simulink model "reconstruct_albatros_dual_15"  (R2021a)
settings: Solver=VariableStepAuto  StartTime=0.0  StopTime=10.0  RelTol=1e-3
undefined symbols (not defined in the file): pfb_coeff_gen_calc
libraries: xbsIndex_r4 x5175, casper_library_misc x31, casper_library_delays x24, xps_library x4
(part 16 of 71)

== system reconstruct_albatros_dual_15/tvg0/tvg ==
  addr : Inport
  data_in : Inport  Port=2
  we : Inport  Port=3
  Terminator : Terminator
  Terminator1 : Terminator
  Terminator2 : Terminator
  calc_add : Subsystem  mask{data_width=64, addr_width=12, sample_rate=sample_rate}
      mask prompts: data_width "data width"; addr_width "address width"; sample_rate "sample rate"
  convert_addr : xbsIndex_r4/Convert  gui_display_data_type=Fixed-point  arith_type=Unsigned  n_bits=addr_width  bin_pt=0  float_type=Single  exp_bits=8  fraction_bits=24  quantization=Truncate  overflow=Wrap  en=off  latency=0  pipeline=off  dbl_ovrd=off  block_type=convert
      settings: xl_area=[0, 0, 0, 0, 0, 0, 0]
  convert_din1 : xbsIndex_r4/Convert  gui_display_data_type=Fixed-point  arith_type=Unsigned  n_bits=64  bin_pt=0  float_type=Single  exp_bits=8  fraction_bits=24  quantization=Truncate  overflow=Wrap  en=off  latency=0  pipeline=off  dbl_ovrd=off  block_type=convert
      settings: xl_area=[0, 0, 0, 0, 0, 0, 0]
  convert_we : xbsIndex_r4/Convert  gui_display_data_type=Fixed-point  arith_type=Unsigned  n_bits=1  bin_pt=0  float_type=Single  exp_bits=8  fraction_bits=24  quantization=Truncate  overflow=Wrap  en=off  latency=0  pipeline=off  dbl_ovrd=off  block_type=convert
      settings: xl_area=[0, 0, 0, 0, 0, 0, 0]
  munge_in : Subsystem  AncestorBlock=casper_library_flow_control/munge  mask(munge){divisions=2, div_size=[32 32], order=[1  0], arith_type_out=Unsigned, bin_pt_out=0}
      mask prompts: divisions "Number of divisions"; div_size "Division size (bits)"; order "Division packing order"; arith_type_out "Output arithmetic type"; bin_pt_out "Output binary point"
      mask help: Splits an input bus into the specified number of divisions and then recombines them in the order specified (most significant division = 0,least = number divisions-1)
      mask init:
      | munge_init(gcb, ...
      |     'divisions', divisions, ...
      |     'div_size', div_size, ...
      |     'order', order, ...
      |     'arith_type_out', arith_type_out, ...
      |     'bin_pt_out', bin_pt_out);
      settings: AttributesFormatString=|
      | split:[32 32]
      | join:[1 0]
      | Unsigned [64,0]
      mask TypeOptions arith_type_out: Unsigned | Signed  (2's comp) | Floating-point
  munge_out : Subsystem  AncestorBlock=casper_library_flow_control/munge  mask(munge){divisions=2, div_size=[32 32], order=[1  0], arith_type_out=Unsigned, bin_pt_out=0}
      mask prompts: divisions "Number of divisions"; div_size "Division size (bits)"; order "Division packing order"; arith_type_out "Output arithmetic type"; bin_pt_out "Output binary point"
      mask help: Splits an input bus into the specified number of divisions and then recombines them in the order specified (most significant division = 0,least = number divisions-1)
      mask init:
      | munge_init(gcb, ...
      |     'divisions', divisions, ...
      |     'div_size', div_size, ...
      |     'order', order, ...
      |     'arith_type_out', arith_type_out, ...
      |     'bin_pt_out', bin_pt_out);
      settings: AttributesFormatString=|
      | split:[32 32]
      | join:[1 0]
      | Unsigned [64,0]
      mask TypeOptions arith_type_out: Unsigned | Signed  (2's comp) | Floating-point
  reconstruct_albatros_dual_15_tvg0_tvg_addr : xbsIndex_r4/Gateway Out  inherit_from_input=off  hdl_port=on  rows=1  columns=1  UseAsDAC=off  DACChannel='1'  interface=None  automatic_assignment=on  address_offset=hex2dec('00')  intf_name=''  intf_description=''  timing_constraint=None  locs_specified=off  LOCs={'A5','B9','A9','C1','A3','G6','E9','A6','A7','A8','B8','B1','B3','D9','B5','B4','B6','C2'}  io_standard={}  block_type=gatewayout
      settings: infoedit="Gateway out block.  Converts Xilinx fixed point inputs into ouputs of type Simulink integer, double, or fixed point.<P><P>Hardware notes:  In hardware these blocks become top level output ports or are discarded, depending on how they are configured."  sginterface={'Nallatech'=>{'xdspkit'=>{'non_memory_mapped_port'=>'uprev_Shared_BRAM_addr'}},'Xilinx'=>{'jtaghwcosim'=>{'non_memory_mapped_port'=>'uprev_Shared_BRAM_addr'},'xdspkit'=>{'non_memory_mapped_port'=>'uprev_Shared_BRAM_addr'}}}  xl_area=[0, 0, 0, 0, 0, 0, 0]
  reconstruct_albatros_dual_15_tvg0_tvg_data_in : xbsIndex_r4/Gateway Out  inherit_from_input=off  hdl_port=on  rows=1  columns=1  UseAsDAC=off  DACChannel='1'  interface=None  automatic_assignment=on  address_offset=hex2dec('00')  intf_name=''  intf_description=''  timing_constraint=None  locs_specified=off  LOCs={'B21','B22','A22','B23','B19','C19','A20','A21','A23','B24','A24','A25','E18','D18','C18','B18'}  io_standard={}  block_type=gatewayout
      settings: infoedit="Gateway out block.  Converts Xilinx fixed point inputs into ouputs of type Simulink integer, double, or fixed point.<P><P>Hardware notes:  In hardware these blocks become top level output ports or are discarded, depending on how they are configured."  sginterface={'Nallatech'=>{'xdspkit'=>{'non_memory_mapped_port'=>'uprev_Shared_BRAM_data_in'}},'Xilinx'=>{'jtaghwcosim'=>{'non_memory_mapped_port'=>'uprev_Shared_BRAM_data_in'},'xdspkit'=>{'non_memory_mapped_port'=>'uprev_Shared_BRAM_data_in'}}}  xl_area=[0, 0, 0, 0, 0, 0, 0]
  reconstruct_albatros_dual_15_tvg0_tvg_data_out : xbsIndex_r4/Gateway In  gui_display_data_type=Fixed-point  arith_type=Unsigned  n_bits=64  bin_pt=0  preci_type=Single  exp_width=8  frac_width=24  rows=1  columns=1  quantization=Truncate  overflow=Wrap  period=sample_rate  UseAsADC=off  ADCChannel='1'  interface=None  automatic_assignment=on  address_offset=hex2dec('00')  intf_name=''  intf_description=''  default_value=0  timing_constraint=None  locs_specified=off  LOCs={}  io_standard={}  inherit_from_input=off  hdl_port=on  dbl_ovrd=off  block_type=gatewayin
      settings: xl_area=[0, 0, 0, 0, 0, 0, 0]
  reconstruct_albatros_dual_15_tvg0_tvg_we : xbsIndex_r4/Gateway Out  inherit_from_input=off  hdl_port=on  rows=1  columns=1  UseAsDAC=off  DACChannel='1'  interface=None  automatic_assignment=on  address_offset=hex2dec('00')  intf_name=''  intf_description=''  timing_constraint=None  locs_specified=off  LOCs={'A14'}  io_standard={}  block_type=gatewayout
      settings: infoedit="Gateway out block.  Converts Xilinx fixed point inputs into ouputs of type Simulink integer, double, or fixed point.<P><P>Hardware notes:  In hardware these blocks become top level output ports or are discarded, depending on how they are configured."  xl_area=[0, 0, 0, 0, 0, 0, 0]
  sim_mem : Subsystem  mask{arith_type=Unsigned, addr_width=12, data_width=64, data_bin_pt=0, init_vals=[0      4294967296      8589934592     12884901888     17179869184     21474836480     25769803776     30064771072     34359738368     38654705664     42949672960     47244640256     51539607552     55834574848     60129542144     64424509440     68719476736     73014444032     77309411328     81604378624     85899345920     90194313216     94489280512     98784247808    103079215104    107374182400    111669149696    115964116992    120259084288    124554051584    128849018880    133143986176    137438953472    141733920768    146028888064    150323855360    154618822656    158913789952    163208757248    167503724544    171798691840    176093659136    180388626432    184683593728    188978561024    193273528320    197568495616    201863462912    206158430208    210453397504    214748364800    219043332096    223338299392    227633266688    231928233984    236223201280    240518168576    244813135872    249108103168    253403070464    257698037760    261993005056    266287972352    270582939648    274877906944    279172874240    283467841536    287762808832    292057776128    296352743424    300647710720    304942678016    309237645312    313532612608    317827579904    322122547200    326417514496    330712481792    335007449088    339302416384    343597383680    347892350976    352187318272    356482285568    360777252864    365072220160    369367187456    373662154752    377957122048    382252089344    386547056640    390842023936    395136991232    399431958528    403726925824    408021893120    412316860416    416611827712    420906795008    425201762304    429496729600    433791696896    438086664192    442381631488    446676598784    450971566080    455266533376    459561500672    463856467968    468151435264    472446402560    476741369856    481036337152    485331304448    489626271744    493921239040    498216206336    502511173632    506806140928    511101108224    515396075520    519691042816    523986010112    528280977408    532575944704    536870912000    541165879296    545460846592    549755813888    554050781184    558345748480    562640715776    566935683072    571230650368    575525617664    579820584960    584115552256    588410519552    592705486848    597000454144    601295421440    605590388736    609885356032    614180323328    618475290624    622770257920    627065225216    631360192512    635655159808    639950127104    644245094400    648540061696    652835028992    657129996288    661424963584    665719930880    670014898176    674309865472    678604832768    682899800064    687194767360    691489734656    695784701952    700079669248    704374636544    708669603840    712964571136    717259538432    721554505728    725849473024    730144440320    734439407616    738734374912    743029342208    747324309504    751619276800    755914244096    760209211392    764504178688    768799145984    773094113280    777389080576    781684047872    785979015168    790273982464    794568949760    798863917056    803158884352    807453851648    811748818944    816043786240    820338753536    824633720832    828928688128    833223655424    837518622720    841813590016    846108557312    850403524608    854698491904    858993459200    863288426496    867583393792    871878361088    876173328384    880468295680    884763262976    889058230272    893353197568    897648164864    901943132160    906238099456    910533066752    914828034048    919123001344    923417968640    927712935936    932007903232    936302870528    940597837824    944892805120    949187772416    953482739712    957777707008    962072674304    966367641600    970662608896    974957576192    979252543488    983547510784    987842478080    992137445376    996432412672   1000727379968   1005022347264   1009317314560   1013612281856   1017907249152   1022202216448   1026497183744   1030792151040   1035087118336   1039382085632   1043677052928   1047972020224   1052266987520   1056561954816   1060856922112   1065151889408   1069446856704 ...(+61534 chars)], sample_rate=1, csp_latency=1}
      mask prompts: arith_type "Output Data Type"; addr_width "Address width"; data_width "Data width"; data_bin_pt "Data Binary Point"; init_vals "Initial values"; sample_rate "Sample rate"; csp_latency "Latency"
      mask init:
      | % set_param([gcb, '/data_to_xilinx'], 'arith_type', arith_type)
      | % set_param([gcb, '/data_to_xilinx'], 'n_bits', get_param(gcb, 'data_width'))
      mask TypeOptions arith_type: Unsigned | Signed  (2's comp)
      mask TypeOptions data_width: 8 | 16 | 32 | 64 | 128
  data_out : Outport  VectorParamsAs1DForOutWhenUnconnected=off
  wires:
  munge_out/1(dout) -> data_out/1
  sim_mem/1(data_out) -> reconstruct_albatros_dual_15_tvg0_tvg_data_out/1
  reconstruct_albatros_dual_15_tvg0_tvg_data_out/1 -> munge_out/1(din)
  convert_addr/1 -> reconstruct_albatros_dual_15_tvg0_tvg_addr/1
  convert_din1/1 -> reconstruct_albatros_dual_15_tvg0_tvg_data_in/1
  data_in/1 -> munge_in/1(din)
  calc_add/1(out) -> convert_addr/1
  reconstruct_albatros_dual_15_tvg0_tvg_we/1 -> Terminator2/1
  reconstruct_albatros_dual_15_tvg0_tvg_data_in/1 -> Terminator1/1
  reconstruct_albatros_dual_15_tvg0_tvg_addr/1 -> Terminator/1
  convert_we/1 -> reconstruct_albatros_dual_15_tvg0_tvg_we/1
  addr/1 -> sim_mem/1(addr), calc_add/1(in)
  we/1 -> sim_mem/3(we), convert_we/1
  munge_in/1(dout) -> sim_mem/2(data), convert_din1/1
